simulink model "FP_Sim"  (R2015a)
settings: Solver=ode45  StartTime=0.0  StopTime=Time  RelTol=1e-3
values from neighbouring files (symbols this model uses):
  Kd = 2    [Theory.m]    (also in Theory_Sim.m)
  Kp = 1    [Theory.m]    (also in Theory_Sim.m)
  TP = 20    [Theory_Sim.m]
undefined symbols (not defined in the file or in its folder): GDen, GNum
settings Model: Creator=Chris  LastModifiedBy=Chris
settings GRTTargetCC: ExtModeTransport=1  ExtModeMexFile=ext_serial_win32_comm  RTWCAPISignals=on  RTWCAPIParams=on

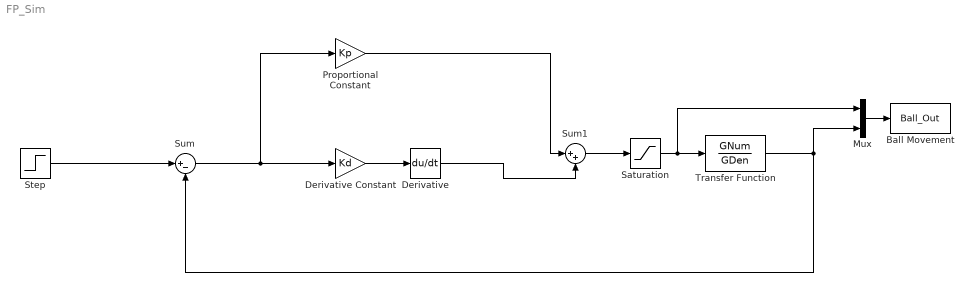
== system FP_Sim ==
  Ball Movement : ToWorkspace  VariableName=Ball_Out  SaveFormat=Timeseries  SampleTime=-1
  Derivative : Derivative
  Derivative Constant : Gain  Gain=Kd
  Mux : Mux  Inputs=2
  Proportional Constant : Gain  Gain=Kp
  Saturation : Saturate  UpperLimit=13  LowerLimit=-13
  Step : Step  Time=0  After=TP  SampleTime=0
  Sum : Sum  Inputs=|+-
  Sum1 : Sum  Inputs=|++
  Transfer Function : TransferFcn  Numerator=GNum  Denominator=GDen
  wires:
  Step/1 -> Sum/1
  Sum/1 -> Proportional Constant/1, Derivative Constant/1
  Derivative Constant/1 -> Derivative/1
  Derivative/1 -> Sum1/2
  Proportional Constant/1 -> Sum1/1
  Transfer Function/1 -> Mux/2, Sum/2
  Saturation/1 -> Mux/1, Transfer Function/1
  Sum1/1 -> Saturation/1
  Mux/1 -> Ball Movement/1
